simulink model "ACRModel"  (Simulink 7.3)
settings: Solver=ode45  StartTime=0.0  StopTime=1920  RelTol=1e-3
undefined symbols (not defined in the file or in its folder): Coef
libraries: simulink x5, dspstat3 x2
settings Model: Creator=admin  LastModifiedBy=admin

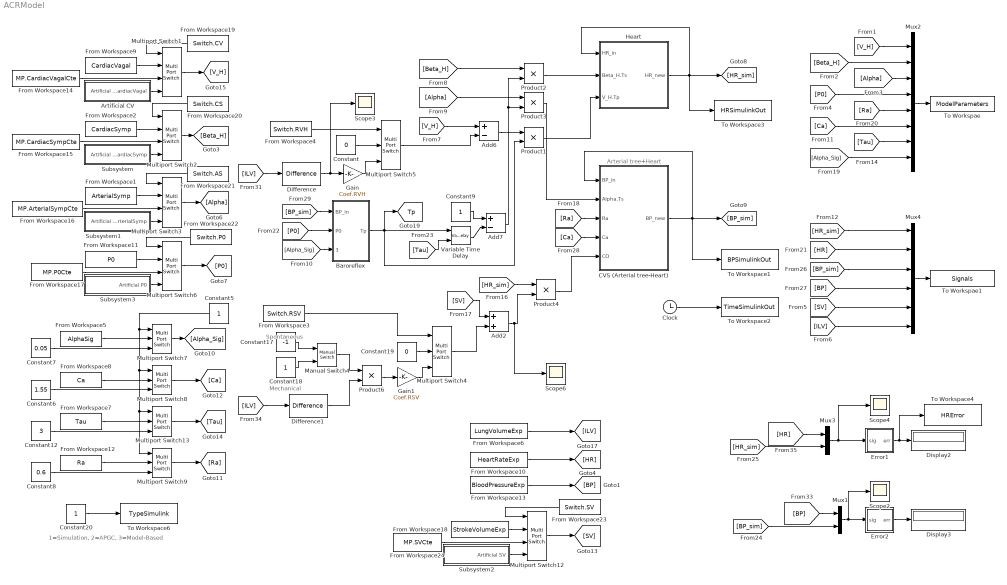
== system ACRModel ==
  note: Arterial tree+Heart
  note: Mechanical
  note: Spontaneous
  note: 1=Simulation,
      | 2=APGC,
      | 3=Model-Based
  Add2 : Sum  OutDataType=fixdt(1, 16)  OutScaling=2^-10
  Add6 : Sum  Inputs=+-  OutDataType=fixdt(1, 16)  OutScaling=2^-10
  Add7 : Sum  Inputs=+-  OutDataType=fixdt(1, 16)  OutScaling=2^-10
  Artificial CV : Subsystem
  Baroreflex : Subsystem
  CVS (Arterial tree-Heart) : Subsystem
  Clock : Clock
      settings: Decimation=10
  Constant : Constant  Value=0  OutDataType=fixdt(1, 16)  OutScaling=2^0
  Constant12 : Constant  Value=3  OutDataType=fixdt(1, 16)  OutScaling=2^0
  Constant17 : Constant  Value=-1  OutDataType=fixdt(1, 16)  OutScaling=2^0
  Constant{5,9,18,20} (4 alike) : Constant  OutDataType=fixdt(1, 16)  OutScaling=2^0
  Constant19 : Constant  Value=0  OutDataType=fixdt(1, 16)  OutScaling=2^0
  Constant6 : Constant  Value=1.55  OutDataType=fixdt(1, 16)  OutScaling=2^0
  Constant7 : Constant  Value=0.05  OutDataType=fixdt(1, 16)  OutScaling=2^0
  Constant8 : Constant  Value=0.6  OutDataType=fixdt(1, 16)  OutScaling=2^0
  Difference : simulink/Discrete/Difference  SystemSampleTime=-1  ICPrevInput=0.0  OutMin=[]  OutMax=[]  OutDataType=fixdt(1, 16)  OutScaling=2^-10  DoSatur=off
  Difference1 : simulink/Discrete/Difference  SystemSampleTime=-1  ICPrevInput=0.0  OutMin=[]  OutMax=[]  OutDataType=fixdt(1, 16)  OutScaling=2^-10  DoSatur=off
  Display2 : Display
  Display3 : Display
  Error1 : Subsystem
  Error2 : Subsystem
  From Workspace1 : FromWorkspace  VariableName=ArterialSymp  SampleTime=1
  From Workspace10 : FromWorkspace  VariableName=HeartRateExp  SampleTime=1
  From Workspace11 : FromWorkspace  VariableName=P0  SampleTime=1
  From Workspace12 : FromWorkspace  VariableName=Ra  SampleTime=0
  From Workspace13 : FromWorkspace  VariableName=BloodPressureExp  SampleTime=1
  From Workspace14 : FromWorkspace  VariableName=MP.CardiacVagalCte  SampleTime=0
  From Workspace15 : FromWorkspace  VariableName=MP.CardiacSympCte  SampleTime=0
  From Workspace16 : FromWorkspace  VariableName=MP.ArterialSympCte  SampleTime=0
  From Workspace17 : FromWorkspace  VariableName=MP.P0Cte  SampleTime=0
  From Workspace18 : FromWorkspace  VariableName=StrokeVolumeExp  SampleTime=1
  From Workspace19 : FromWorkspace  VariableName=Switch.CV  SampleTime=0
  From Workspace2 : FromWorkspace  VariableName=CardiacSymp  SampleTime=1
  From Workspace20 : FromWorkspace  VariableName=Switch.CS  SampleTime=0
  From Workspace21 : FromWorkspace  VariableName=Switch.AS  SampleTime=0
  From Workspace22 : FromWorkspace  VariableName=Switch.P0  SampleTime=0
  From Workspace23 : FromWorkspace  VariableName=Switch.SV  SampleTime=0
  From Workspace24 : FromWorkspace  VariableName=MP.SVCte  SampleTime=0
  From Workspace3 : FromWorkspace  VariableName=Switch.RSV  SampleTime=0
  From Workspace4 : FromWorkspace  VariableName=Switch.RVH  SampleTime=0
  From Workspace5 : FromWorkspace  VariableName=AlphaSig  SampleTime=0
  From Workspace6 : FromWorkspace  VariableName=LungVolumeExp  SampleTime=1
  From Workspace7 : FromWorkspace  VariableName=Tau  SampleTime=0
  From Workspace8 : FromWorkspace  VariableName=Ca  SampleTime=0
  From Workspace9 : FromWorkspace  VariableName=CardiacVagal  SampleTime=1
  Gain : Gain  Gain=Coef.RVH  ParameterDataType=fixdt(1, 16)  ParameterScaling=2^0  OutDataType=fixdt(1, 16)  OutScaling=2^0
  Gain1 : Gain  Gain=Coef.RSV  ParameterDataType=fixdt(1, 16)  ParameterScaling=2^0  OutDataType=fixdt(1, 16)  OutScaling=2^0
  Heart : Subsystem
  Manual Switch4 : simulink/Signal Routing/Manual Switch  SystemSampleTime=-1  sw=0  action=0  varsize=off
  Multiport Switch{1..3,6,12} (5 alike) : MultiPortSwitch  OutDataType=fixdt(1, 16)  OutScaling=2^0
  Multiport Switch{4..5,7..9,13} (6 alike) : MultiPortSwitch  Inputs=2  OutDataType=fixdt(1, 16)  OutScaling=2^0
  Mux1 : Mux  Inputs=2
  Mux2 : Mux  Inputs=8
  Mux3 : Mux  Inputs=2
  Mux4 : Mux  Inputs=6
  Product{1..4,6} (5 alike) : Product  OutDataType=fixdt(1, 16)  OutScaling=2^0  RndMeth=Zero
  Scope{2..4,6} (4 alike) : Scope
      Scope2 settings: YMin=67.5  YMax=125
      Scope3 settings: YMin=1  YMax=1.95  SaveName=ScopeData3
      Scope4 settings: YMin=1  YMax=1.95  SaveName=ScopeData2
      Scope6 settings: YMin=97.75  YMax=101  SaveName=ScopeData5
  Subsystem : Subsystem
  Subsystem1 : Subsystem
  Subsystem2 : Subsystem
  Subsystem3 : Subsystem
  To Workspace1 : ToWorkspace  VariableName=BPSimulinkOut  SampleTime=-1  SaveFormat=Structure
  To Workspace2 : ToWorkspace  VariableName=TimeSimulinkOut  SampleTime=-1  SaveFormat=Structure
  To Workspace3 : ToWorkspace  VariableName=HRSimulinkOut  SampleTime=-1  SaveFormat=Structure
  To Workspace4 : ToWorkspace  VariableName=HRError  SampleTime=-1  SaveFormat=Structure
  To Workspace6 : ToWorkspace  VariableName=TypeSimulink  SampleTime=-1  SaveFormat=Structure
  To Workspae : ToWorkspace  VariableName=ModelParameters  SampleTime=-1  SaveFormat=Structure
  To Workspae1 : ToWorkspace  VariableName=Signals  SampleTime=-1  SaveFormat=Structure
  Variable Time Delay : VariableTransportDelay  MaximumDelay=10
  tag scope: Tp=global
  wires:
  From Workspace5/1 -> Multiport Switch7/2
  From Workspace8/1 -> Multiport Switch8/2
  From Workspace12/1 -> Multiport Switch9/2
  Multiport Switch7/1 -> [Alpha_Sig]
  Multiport Switch8/1 -> [Ca]
  Multiport Switch9/1 -> [Ra]
  Constant6/1 -> Multiport Switch8/3
  Constant7/1 -> Multiport Switch7/3
  Constant8/1 -> Multiport Switch9/3
  Constant5/1 -> Multiport Switch7/1, Multiport Switch8/1, Multiport Switch13/1, Multiport Switch9/1
  Baroreflex/1(Tp) -> Product1/2, Variable Time Delay/1, [Tp]
  Constant9/1 -> Add7/1
  Product2/1 -> Heart/2(Beta_H.Ts)
  Product1/1 -> Heart/3(V_H.Tp)
  Heart/1(HR_new) -> [HR_sim], Heart/1(HR_in), To Workspace3/1
  Product3/1 -> CVS (Arterial tree-Heart)/2(Alpha.Ts)
  [Ra] -> CVS (Arterial tree-Heart)/3(Ra)
  [Ca] -> CVS (Arterial tree-Heart)/4(Ca)
  Add7/1 -> Product3/2, Product2/2
  [Beta_H] -> Product2/1
  [Alpha] -> Product3/1
  [BP_sim] -> Baroreflex/1(BP_in)
  [P0] -> Baroreflex/2(P0)
  CVS (Arterial tree-Heart)/1(BP_new) -> [BP_sim], CVS (Arterial tree-Heart)/1(BP_in), To Workspace1/1
  [Alpha_Sig] -> Baroreflex/3(Alpha_Sig)
  Variable Time Delay/1 -> Add7/2
  [Tau] -> Variable Time Delay/2
  From Workspace7/1 -> Multiport Switch13/2
  Multiport Switch13/1 -> [Tau]
  Constant12/1 -> Multiport Switch13/3
  [ILV] -> Difference/1
  Gain/1 -> Multiport Switch5/3
  Constant/1 -> Multiport Switch5/2
  [V_H] -> Add6/1
  Multiport Switch5/1 -> Add6/2
  Add6/1 -> Product1/1
  From Workspace10/1 -> [HR]
  From Workspace13/1 -> [BP]
  From Workspace6/1 -> [ILV]
  From Workspace18/1 -> Multiport Switch12/2
  From Workspace24/1 -> Multiport Switch12/3
  From Workspace23/1 -> Multiport Switch12/1
  Multiport Switch12/1 -> [SV]
  Mux1/1 -> Scope2/1, Error2/1(sig)
  Error2/1(err) -> Display3/1
  Mux3/1 -> Error1/1(sig), Scope4/1
  Error1/1(err) -> Display2/1, To Workspace4/1
  [HR] -> Mux3/1
  [BP] -> Mux1/1
  [BP_sim] -> Mux1/2
  Multiport Switch6/1 -> [P0]
  Multiport Switch3/1 -> [Alpha]
  Multiport Switch2/1 -> [Beta_H]
  Multiport Switch1/1 -> [V_H]
  From Workspace9/1 -> Multiport Switch1/2
  From Workspace2/1 -> Multiport Switch2/2
  From Workspace1/1 -> Multiport Switch3/2
  From Workspace11/1 -> Multiport Switch6/2
  From Workspace14/1 -> Multiport Switch1/3
  From Workspace15/1 -> Multiport Switch2/3
  From Workspace16/1 -> Multiport Switch3/3
  From Workspace19/1 -> Multiport Switch1/1
  From Workspace20/1 -> Multiport Switch2/1
  From Workspace21/1 -> Multiport Switch3/1
  From Workspace22/1 -> Multiport Switch6/1
  Artificial CV/1(Artificial CardiacVagal) -> Multiport Switch1/4
  Subsystem/1(Artificial CardiacSymp) -> Multiport Switch2/4
  Subsystem1/1(Artificial ArterialSymp) -> Multiport Switch3/4
  Subsystem3/1(Artificial P0) -> Multiport Switch6/4
  Subsystem2/1(Artificial SV) -> Multiport Switch12/4
  Product4/1 -> CVS (Arterial tree-Heart)/5(CO)
  [HR_sim] -> Product4/1
  [SV] -> Add2/1
  Add2/1 -> Product4/2, Scope6/1
  Constant17/1 -> Manual Switch4/1
  Constant18/1 -> Manual Switch4/2
  Manual Switch4/1 -> Product6/1
  Product6/1 -> Gain1/1
  Multiport Switch4/1 -> Add2/2
  Constant19/1 -> Multiport Switch4/2
  [ILV] -> Difference1/1
  Gain1/1 -> Multiport Switch4/3
  Mux2/1 -> To Workspae/1
  [V_H] -> Mux2/1
  [Beta_H] -> Mux2/2
  [Alpha] -> Mux2/3
  [P0] -> Mux2/4
  [Ca] -> Mux2/6
  [Tau] -> Mux2/7
  [Alpha_Sig] -> Mux2/8
  [Ra] -> Mux2/5
  [HR_sim] -> Mux4/1
  [HR] -> Mux4/2
  [BP_sim] -> Mux4/3
  [BP] -> Mux4/4
  [SV] -> Mux4/5
  [ILV] -> Mux4/6
  Mux4/1 -> To Workspae1/1
  Difference/1 -> Gain/1, Scope3/1
  Difference1/1 -> Product6/2
  [HR_sim] -> Mux3/2
  Clock/1 -> To Workspace2/1
  Constant20/1 -> To Workspace6/1
  From Workspace3/1 -> Multiport Switch4/1
  From Workspace4/1 -> Multiport Switch5/1
  From Workspace17/1 -> Multiport Switch6/3

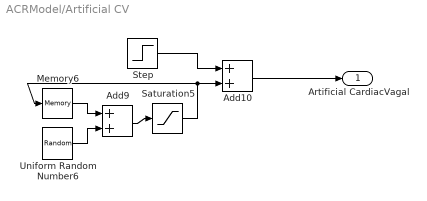
== system ACRModel/Artificial CV ==
  Add10 : Sum  OutDataType=fixdt(1, 16)  OutScaling=2^-10
  Add9 : Sum  OutDataType=fixdt(1, 16)  OutScaling=2^-10
  Memory6 : Memory  X0=1.17  InheritSampleTime=on  LinearizeAsDelay=on
  Saturation5 : Saturate  UpperLimit=2.24  LowerLimit=0.58  OutDataType=fixdt(1, 16)  OutScaling=2^0
  Step : Step  Time=500  After=0.5  SampleTime=0
  Uniform Random Number6 : UniformRandomNumber  Minimum=-0.025  Maximum=0.025  SampleTime=10
  Artificial CardiacVagal : Outport
  wires:
  Add9/1 -> Saturation5/1
  Uniform Random Number6/1 -> Add9/2
  Memory6/1 -> Add9/1
  Saturation5/1 -> Memory6/1, Add10/2
  Step/1 -> Add10/1
  Add10/1 -> Artificial CardiacVagal/1

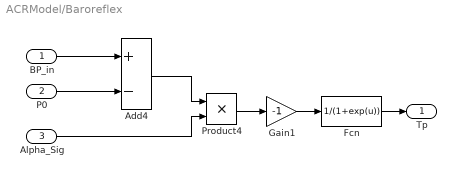
== system ACRModel/Baroreflex ==
  BP_in : Inport
  P0 : Inport  Port=2
  Alpha_Sig : Inport  Port=3
  Add4 : Sum  Inputs=+-  OutDataType=fixdt(1, 16)  OutScaling=2^-10
  Fcn : Fcn  Expr=1/(1+exp(u))
  Gain1 : Gain  Gain=-1  ParameterDataType=fixdt(1, 16)  ParameterScaling=2^0  OutDataType=fixdt(1, 16)  OutScaling=2^0
  Product4 : Product  OutDataType=fixdt(1, 16)  OutScaling=2^0  RndMeth=Zero
  Tp : Outport
  wires:
  Add4/1 -> Product4/1
  Gain1/1 -> Fcn/1
  Product4/1 -> Gain1/1
  BP_in/1 -> Add4/1
  Fcn/1 -> Tp/1
  Alpha_Sig/1 -> Product4/2
  P0/1 -> Add4/2

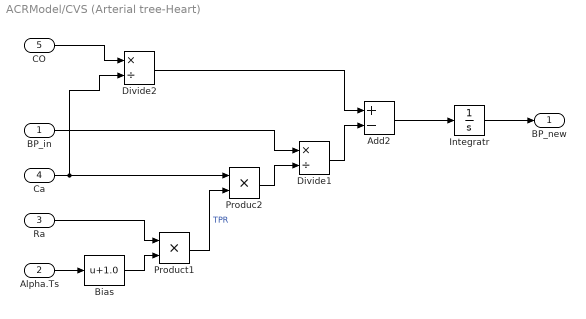
== system ACRModel/CVS (Arterial tree-Heart) ==
  BP_in : Inport
  Alpha.Ts : Inport  Port=2
  Ra : Inport  Port=3
  Ca : Inport  Port=4
  CO : Inport  Port=5
  Add2 : Sum  Inputs=+-  OutDataType=fixdt(1, 16)  OutScaling=2^-10
  Bias : Bias  Bias=1.0
  Divide1 : Product  Inputs=*/  OutDataType=fixdt(1, 16)  OutScaling=2^-10
  Divide2 : Product  Inputs=*/  OutDataType=fixdt(1, 16)  OutScaling=2^-10
  Integratr : Integrator  InitialCondition=100
  Produc2 : Product  OutDataType=fixdt(1, 16)  OutScaling=2^0  RndMeth=Zero
  Product1 : Product  OutDataType=fixdt(1, 16)  OutScaling=2^0  RndMeth=Zero
  BP_new : Outport
  wires:
  Add2/1 -> Integratr/1
  BP_in/1 -> Divide1/1
  Integratr/1 -> BP_new/1
  Divide2/1 -> Add2/1
  CO/1 -> Divide2/1
  Product1/1 -> Produc2/2  "TPR"
  Bias/1 -> Product1/2
  Ra/1 -> Product1/1
  Alpha.Ts/1 -> Bias/1
  Divide1/1 -> Add2/2
  Produc2/1 -> Divide1/2
  Ca/1 -> Produc2/1, Divide2/2

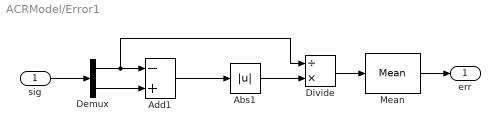
== system ACRModel/Error1 ==
  sig : Inport
  Abs1 : Abs  OutDataType=fixdt(1, 16)  OutScaling=2^0
  Add1 : Sum  Inputs=-+  OutDataType=fixdt(1, 16)  OutScaling=2^-10
  Demux : Demux  Outputs=2
  Divide : Product  Inputs=/*  OutDataType=fixdt(1, 16)  OutScaling=2^-10
  Mean : dspstat3/Mean  DialogController=dspDDGCreate  DialogControllerArgs=DataTag0  run=off  reset_popup=None  directionMode=Each column  dimension=1  treatSBRowAsCol=on  roiEnable=off  roiType=Rectangles  roiPortion=Entire ROI  roiOutput=Individual statistics for each ROI  roiFlag=off  roundingMode=Floor  overflowMode=off
  err : Outport
  wires:
  sig/1 -> Demux/1
  Mean/1 -> err/1
  Divide/1 -> Mean/1
  Abs1/1 -> Divide/2
  Demux/2 -> Add1/2
  Demux/1 -> Divide/1, Add1/1
  Add1/1 -> Abs1/1

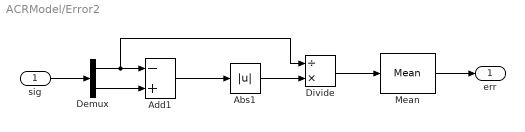
== system ACRModel/Error2 ==
  sig : Inport
  Abs1 : Abs  OutDataType=fixdt(1, 16)  OutScaling=2^0
  Add1 : Sum  Inputs=-+  OutDataType=fixdt(1, 16)  OutScaling=2^-10
  Demux : Demux  Outputs=2
  Divide : Product  Inputs=/*  OutDataType=fixdt(1, 16)  OutScaling=2^-10
  Mean : dspstat3/Mean  DialogController=dspDDGCreate  DialogControllerArgs=DataTag1  run=off  reset_popup=None  directionMode=Each column  dimension=1  treatSBRowAsCol=on  roiEnable=off  roiType=Rectangles  roiPortion=Entire ROI  roiOutput=Individual statistics for each ROI  roiFlag=off  roundingMode=Floor  overflowMode=off
  err : Outport
  wires:
  Add1/1 -> Abs1/1
  Demux/1 -> Add1/1, Divide/1
  Demux/2 -> Add1/2
  Abs1/1 -> Divide/2
  Divide/1 -> Mean/1
  Mean/1 -> err/1
  sig/1 -> Demux/1

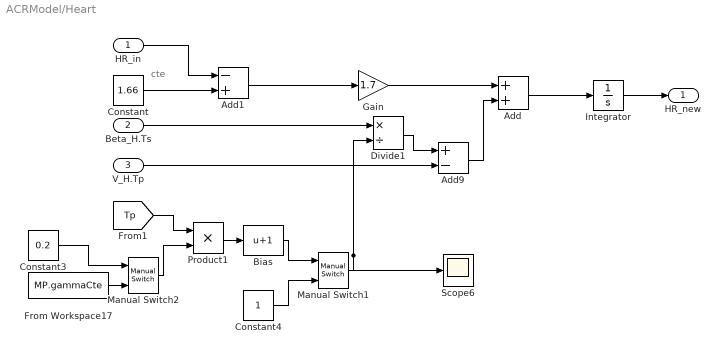
== system ACRModel/Heart ==
  note: cte
  HR_in : Inport
  Beta_H.Ts : Inport  Port=2
  V_H.Tp : Inport  Port=3
  Add : Sum  OutDataType=fixdt(1, 16)  OutScaling=2^-10
  Add1 : Sum  Inputs=-+  OutDataType=fixdt(1, 16)  OutScaling=2^-10
  Add9 : Sum  Inputs=+-  OutDataType=fixdt(1, 16)  OutScaling=2^-10
  Bias : Bias  Bias=1
  Constant : Constant  Value=1.66  OutDataType=fixdt(1, 16)  OutScaling=2^0
  Constant3 : Constant  Value=0.2  OutDataType=fixdt(1, 16)  OutScaling=2^0
  Constant4 : Constant  OutDataType=fixdt(1, 16)  OutScaling=2^0
  Divide1 : Product  Inputs=*/  OutDataType=fixdt(1, 16)  OutScaling=2^-10
  From Workspace17 : FromWorkspace  VariableName=MP.gammaCte  SampleTime=0
  Gain : Gain  Gain=1.7  ParameterDataType=fixdt(1, 16)  ParameterScaling=2^0  OutDataType=fixdt(1, 16)  OutScaling=2^0
  Integrator : Integrator  InitialCondition=1
  Manual Switch1 : simulink/Signal Routing/Manual Switch  SystemSampleTime=-1  sw=1  action=0  varsize=off
  Manual Switch2 : simulink/Signal Routing/Manual Switch  SystemSampleTime=-1  sw=1  action=0  varsize=off
  Product1 : Product  OutDataType=fixdt(1, 16)  OutScaling=2^0  RndMeth=Zero
  Scope6 : Scope
      settings: YMin=97.75  YMax=101  SaveName=ScopeData6
  HR_new : Outport
  wires:
  Constant/1 -> Add1/2
  Add1/1 -> Gain/1
  Gain/1 -> Add/1
  HR_in/1 -> Add1/1
  Add/1 -> Integrator/1
  Add9/1 -> Add/2
  [Tp] -> Product1/1
  Product1/1 -> Bias/1
  Beta_H.Ts/1 -> Divide1/1
  Divide1/1 -> Add9/1
  V_H.Tp/1 -> Add9/2
  Bias/1 -> Manual Switch1/1
  Manual Switch1/1 -> Divide1/2, Scope6/1
  Constant4/1 -> Manual Switch1/2
  Integrator/1 -> HR_new/1
  Manual Switch2/1 -> Product1/2
  From Workspace17/1 -> Manual Switch2/2
  Constant3/1 -> Manual Switch2/1

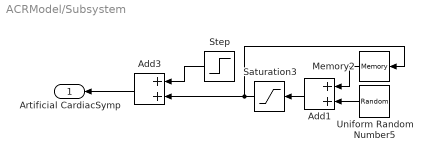
== system ACRModel/Subsystem ==
  Add1 : Sum  OutDataType=fixdt(1, 16)  OutScaling=2^-10
  Add3 : Sum  OutDataType=fixdt(1, 16)  OutScaling=2^-10
  Memory2 : Memory  X0=0.84  InheritSampleTime=on  LinearizeAsDelay=on
  Saturation3 : Saturate  UpperLimit=1.68  LowerLimit=0.42  OutDataType=fixdt(1, 16)  OutScaling=2^0
  Step : Step  Time=500  After=0.5  SampleTime=0
  Uniform Random Number5 : UniformRandomNumber  Minimum=-0.025  Maximum=0.025  Seed=1  SampleTime=10
  Artificial CardiacSymp : Outport
  wires:
  Memory2/1 -> Add1/1
  Uniform Random Number5/1 -> Add1/2
  Add1/1 -> Saturation3/1
  Saturation3/1 -> Memory2/1, Add3/2
  Step/1 -> Add3/1
  Add3/1 -> Artificial CardiacSymp/1

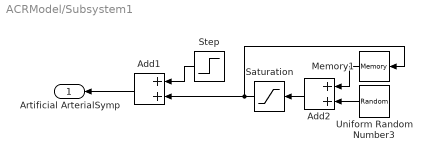
== system ACRModel/Subsystem1 ==
  Add1 : Sum  OutDataType=fixdt(1, 16)  OutScaling=2^-10
  Add2 : Sum  OutDataType=fixdt(1, 16)  OutScaling=2^-10
  Memory1 : Memory  X0=1.3  InheritSampleTime=on  LinearizeAsDelay=on
  Saturation : Saturate  UpperLimit=2.6  LowerLimit=0.65  OutDataType=fixdt(1, 16)  OutScaling=2^0
  Step : Step  Time=500  After=0.5  SampleTime=0
  Uniform Random Number3 : UniformRandomNumber  Minimum=-0.025  Maximum=0.025  Seed=2  SampleTime=10
  Artificial ArterialSymp : Outport
  wires:
  Memory1/1 -> Add2/1
  Uniform Random Number3/1 -> Add2/2
  Add2/1 -> Saturation/1
  Saturation/1 -> Memory1/1, Add1/2
  Step/1 -> Add1/1
  Add1/1 -> Artificial ArterialSymp/1

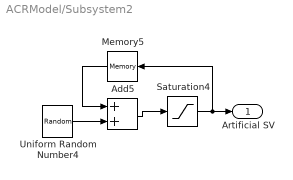
== system ACRModel/Subsystem2 ==
  Add5 : Sum  OutDataType=fixdt(1, 16)  OutScaling=2^-10
  Memory5 : Memory  X0=1.3
  Saturation4 : Saturate  UpperLimit=100  LowerLimit=25  OutDataType=fixdt(1, 16)  OutScaling=2^0
  Uniform Random Number4 : UniformRandomNumber  Minimum=-0.1  Maximum=0.1  SampleTime=500
  Artificial SV : Outport
  wires:
  Memory5/1 -> Add5/1
  Uniform Random Number4/1 -> Add5/2
  Add5/1 -> Saturation4/1
  Saturation4/1 -> Memory5/1, Artificial SV/1

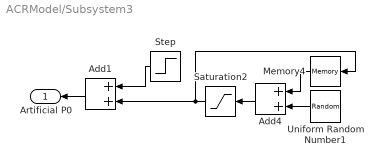
== system ACRModel/Subsystem3 ==
  Add1 : Sum  OutDataType=fixdt(1, 16)  OutScaling=2^-10
  Add4 : Sum  OutDataType=fixdt(1, 16)  OutScaling=2^-10
  Memory4 : Memory  X0=100  InheritSampleTime=on  LinearizeAsDelay=on
  Saturation2 : Saturate  UpperLimit=200  LowerLimit=50  OutDataType=fixdt(1, 16)  OutScaling=2^0
  Step : Step  Time=500  After=30  SampleTime=0
  Uniform Random Number1 : UniformRandomNumber  Minimum=-5  Maximum=5  SampleTime=20
  Artificial P0 : Outport
  wires:
  Memory4/1 -> Add4/1
  Uniform Random Number1/1 -> Add4/2
  Add4/1 -> Saturation2/1
  Saturation2/1 -> Memory4/1, Add1/2
  Step/1 -> Add1/1
  Add1/1 -> Artificial P0/1
